simulink model "ejercicio3"  (R2024b)
settings: Solver=VariableStepAuto  StartTime=0.0  StopTime=5  RelTol=1e-3
settings Model: Creator=david.andrino  LastModifiedBy=david
settings DataIOCC: ReturnWorkspaceOutputs=off
settings RTWCC: GPUComputeCapability=3.5

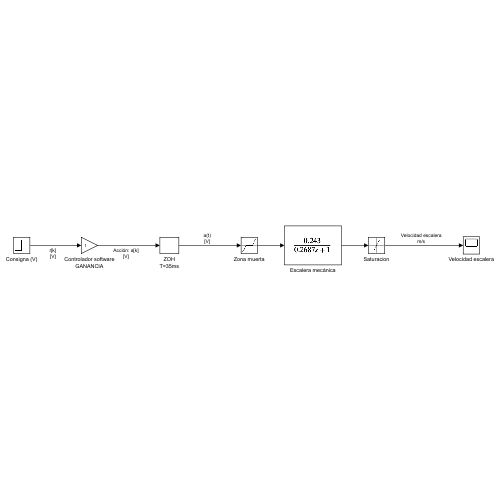
[thumbnail: Simulink's stored preview of the top-level diagram]
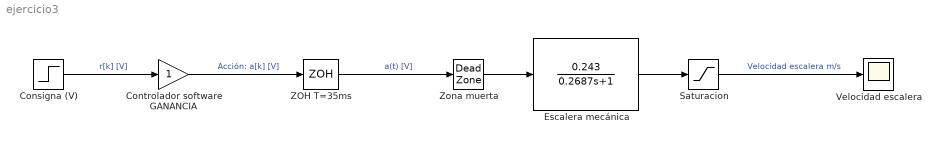
== system ejercicio3 ==
  Consigna (V) : Step  Time=0  SampleTime=0
  Controlador software GANANCIA : Gain
  Escalera mecánica : TransferFcn  Numerator=0.243  Denominator=[0.2687 1]
  Saturacion : Saturate  UpperLimit=2.11  LowerLimit=-2.11
  Velocidad escalera : Scope
  ZOH T=35ms : ZeroOrderHold  SampleTime=35e-3
  Zona muerta : DeadZone  LowerValue=-0.19  UpperValue=0.21
  wires:
  Consigna (V)/1 -> Controlador software GANANCIA/1  "r[k] [V]"
  Controlador software GANANCIA/1 -> ZOH T=35ms/1  "Acción: a[k] [V]"
  ZOH T=35ms/1 -> Zona muerta/1  "a(t) [V]"
  Saturacion/1 -> Velocidad escalera/1  "Velocidad escalera m/s"
  Zona muerta/1 -> Escalera mecánica/1
  Escalera mecánica/1 -> Saturacion/1
